simulink model "Gyro_Sensor_SensorProcessing_Test"  (R2018b)
settings: Solver=VariableStepAuto  StartTime=0.0  StopTime=1  RelTol=1e-3
libraries: gyroscope_lib x3, maggyroProcessing_lib x1
settings Model: Creator=Nick's PC  LastModifiedBy=Taylor

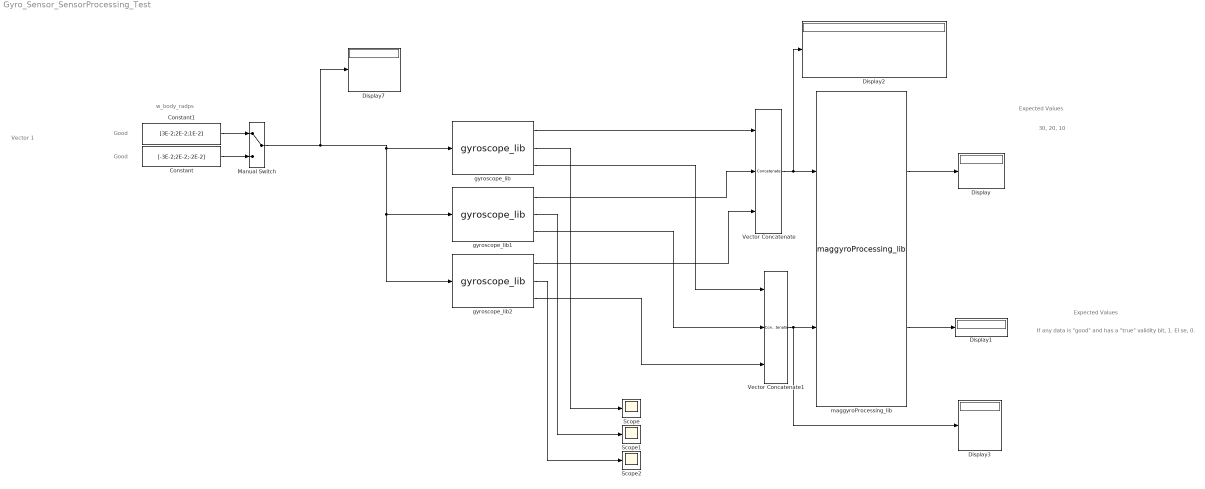
== system Gyro_Sensor_SensorProcessing_Test ==
  note: Expected Values
  note: Good
  note: Expected Values
  note: Good
  note: Vector 1
  note: w_body_radps
  note: If any data is "good" and has a "true" validity bit, 1. El se, 0.
  note: 30, 20, 10
  Constant : Constant  Value=[-3E-2;2E-2;-2E-2]
  Constant1 : Constant  Value=[3E-2;2E-2;1E-2]
  Display{,1..3,7} (5 alike) : Display
  Manual Switch : ManualSwitch
  Scope : Scope
  Scope1 : Scope
  Scope2 : Scope
  Vector Concatenate : Concatenate  NumInputs=3  Mode=Multidimensional array  ConcatenateDimension=2
  Vector Concatenate1 : Concatenate  NumInputs=3  ConcatenateDimension=2
  gyroscope_lib : gyroscope_lib/gyroscope_lib  id_s=1
  gyroscope_lib1 : gyroscope_lib/gyroscope_lib  id_s=2
  gyroscope_lib2 : gyroscope_lib/gyroscope_lib  id_s=3
  maggyroProcessing_lib : maggyroProcessing_lib/maggyroProcessing_lib  static_range_max_value=fswParams.sensors.gyro_static_range  offset_calibration_matrix=fswParams.sensors.gyro_offset  max_err=fswParams.sensors.gyro_max_err  rotation_calibration_matrix=fswParams.sensors.gyro_rotate  Gain=1
  wires:
  Constant1/1 -> Manual Switch/1
  maggyroProcessing_lib/1 -> Display/1
  Constant/1 -> Manual Switch/2
  Manual Switch/1 -> Display7/1, gyroscope_lib2/1, gyroscope_lib1/1, gyroscope_lib/1
  Vector Concatenate/1 -> Display2/1, maggyroProcessing_lib/1
  Vector Concatenate1/1 -> maggyroProcessing_lib/2, Display3/1
  maggyroProcessing_lib/2 -> Display1/1
  gyroscope_lib/1 -> Vector Concatenate/1
  gyroscope_lib1/1 -> Vector Concatenate/2
  gyroscope_lib2/1 -> Vector Concatenate/3
  gyroscope_lib2/3 -> Vector Concatenate1/3
  gyroscope_lib1/3 -> Vector Concatenate1/2
  gyroscope_lib/3 -> Vector Concatenate1/1
  gyroscope_lib2/2 -> Scope2/1
  gyroscope_lib1/2 -> Scope1/1
  gyroscope_lib/2 -> Scope/1
